simulink model "wind_generation"  (R2024b)
settings: Solver=VariableStepAuto  StartTime=0.0  StopTime=143  RelTol=1e-3
undefined symbols (not defined in the file): F, Light, MIL
libraries: aerolibwind2 x5
settings Model: Creator=Utilizador  LastModifiedBy=Utilizador
settings DebuggingCC: SignalInfNanChecking=warning

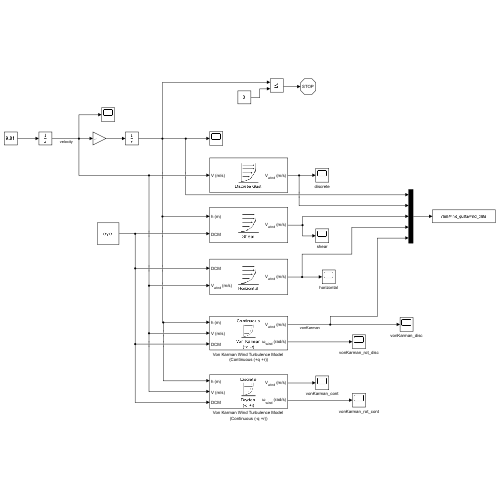
[thumbnail: Simulink's stored preview of the top-level diagram]
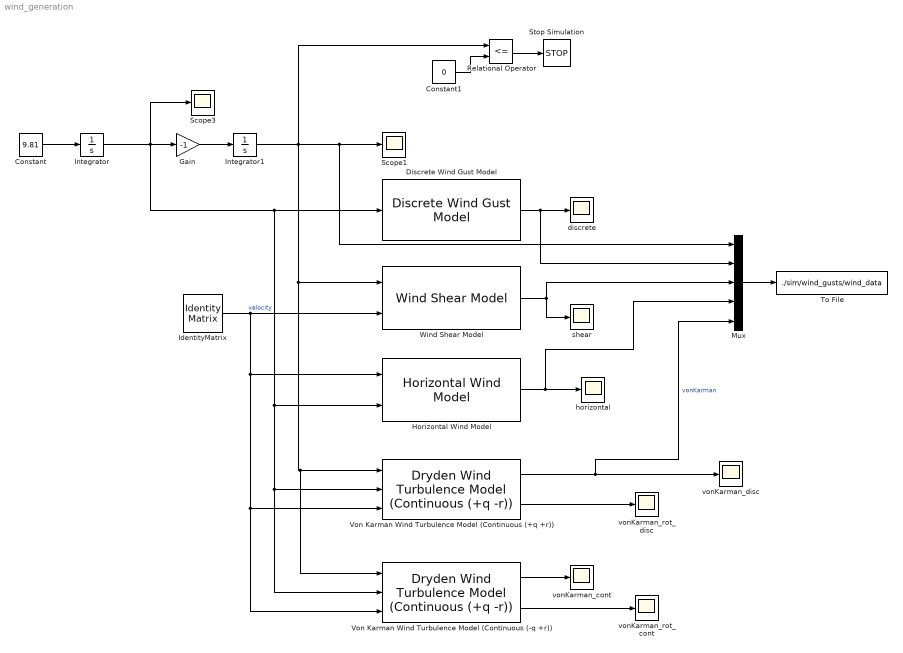
== system wind_generation ==
  Constant : Constant  Value=9.81
  Constant1 : Constant  Value=0
  Discrete Wind Gust Model : aerolibwind2/Discrete Wind Gust Model  units=Metric (MKS)  Gx=on  Gy=on  Gz=on  t_0=5  d_m=[120 120 80]  v_m=[3.5 3.5 3.0]
  Gain : Gain  Gain=-1
  Horizontal Wind Model : aerolibwind2/Horizontal Wind Model  units=Metric (MKS)  Vw_source=External  Vwind=15  W_source=Internal  Wdeg=60
  IdentityMatrix : IdentityMatrix  OutputDimensions=3
  Integrator : Integrator  InitialCondition=1
  Integrator1 : Integrator  InitialCondition=25000
  Mux : Mux  Inputs=5
  Relational Operator : RelationalOperator  Operator=<=  OutDataTypeStr=boolean  RndMeth=Simplest  InputSameDT=off
  Scope1 : Scope
  Scope3 : Scope
  Stop Simulation : Stop
  To File : ToFile  Filename=./sim/wind_gusts/wind_data
  Von Karman Wind Turbulence Model (Continuous (+q +r)) : aerolibwind2/Dryden Wind Turbulence Model  (Continuous (+q -r))  units=Metric (MKS)  spec=MIL-F-8785C  model=Continuous Von Karman (+q -r)  W20=15  Wdeg=0  TurbProb=10^-2 - Light  L_high=762  Wingspan=10  ts=0.1  Seed=[23341 23342 23343 23344]  T_on=on
      settings: LibrarySourceBlock=|
      | aerolibwind2/Von Karman Wind Turbulence Model
      | (Continuous (+q +r))
  Von Karman Wind Turbulence Model (Continuous (-q +r)) : aerolibwind2/Dryden Wind Turbulence Model  (Continuous (+q -r))  units=Metric (MKS)  spec=MIL-F-8785C  model=Discrete Dryden (-q +r)  W20=15  Wdeg=0  TurbProb=10^-2 - Light  L_high=762  Wingspan=10  ts=0.1  Seed=[23341 23342 23343 23344]  T_on=on
      settings: LibrarySourceBlock=|
      | aerolibwind2/Von Karman Wind Turbulence Model
      | (Continuous (-q +r))
  Wind Shear Model : aerolibwind2/Wind Shear Model  units=Metric (MKS)  phase=Category C - Terminal Flight Phase  W_20=15  Wdeg=45
  discrete : Scope
  horizontal : Scope
  shear : Scope
  vonKarman_cont : Scope
  vonKarman_disc : Scope
  vonKarman_rot_cont : Scope
  vonKarman_rot_disc : Scope
  wires:
  Integrator1/1 -> Relational Operator/1, Mux/1, Scope1/1, Wind Shear Model/1, Von Karman Wind Turbulence Model (Continuous (-q +r))/1, Von Karman Wind Turbulence Model (Continuous (+q +r))/1
  Integrator/1 -> Gain/1, Scope3/1, Horizontal Wind Model/2, Von Karman Wind Turbulence Model (Continuous (-q +r))/2, Von Karman Wind Turbulence Model (Continuous (+q +r))/2, Discrete Wind Gust Model/1  "velocity"
  Discrete Wind Gust Model/1 -> Mux/2, discrete/1
  IdentityMatrix/1 -> Wind Shear Model/2, Von Karman Wind Turbulence Model (Continuous (-q +r))/3, Von Karman Wind Turbulence Model (Continuous (+q +r))/3, Horizontal Wind Model/1
  Wind Shear Model/1 -> Mux/3, shear/1
  Horizontal Wind Model/1 -> horizontal/1, Mux/4
  Relational Operator/1 -> Stop Simulation/1
  Constant1/1 -> Relational Operator/2
  Von Karman Wind Turbulence Model (Continuous (+q +r))/1 -> Mux/5, vonKarman_disc/1  "vonKarman"
  Gain/1 -> Integrator1/1
  Constant/1 -> Integrator/1
  Von Karman Wind Turbulence Model (Continuous (+q +r))/2 -> vonKarman_rot_disc/1
  Von Karman Wind Turbulence Model (Continuous (-q +r))/1 -> vonKarman_cont/1
  Von Karman Wind Turbulence Model (Continuous (-q +r))/2 -> vonKarman_rot_cont/1
  Mux/1 -> To File/1
